simulink model "PMSM_CascadedMPC"  (R2025b)
settings: Solver=ode3  StartTime=0.0  StopTime=12  FixedStep=5e-6  MaxStep=1e-4  RelTol=1e-3
PreLoadFcn:
  | run('params_pmsm_inverter')
undefined symbols (not defined in the file): B_fric, J, Ld, Lq, pp, PsiPM, Rs, Ts_ctrl, Ts_sim, Vdc
libraries: nesl_utility x16, fl_lib x11, ee_lib x8, simulink x1, sdl_lib x1
(part 1 of 2)
settings Model: SimulationMode=accelerator  Creator=Harish  LastModifiedBy=Harish

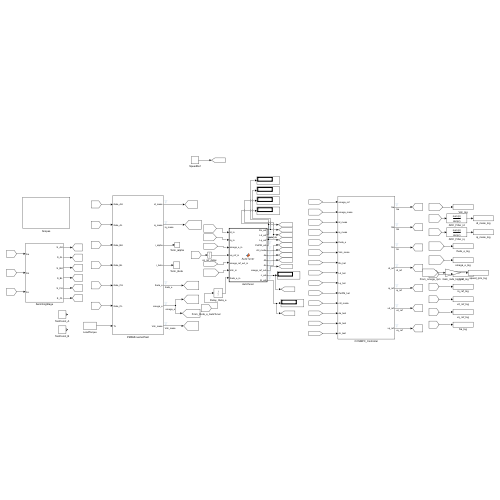
[thumbnail: Simulink's stored preview of the top-level diagram]
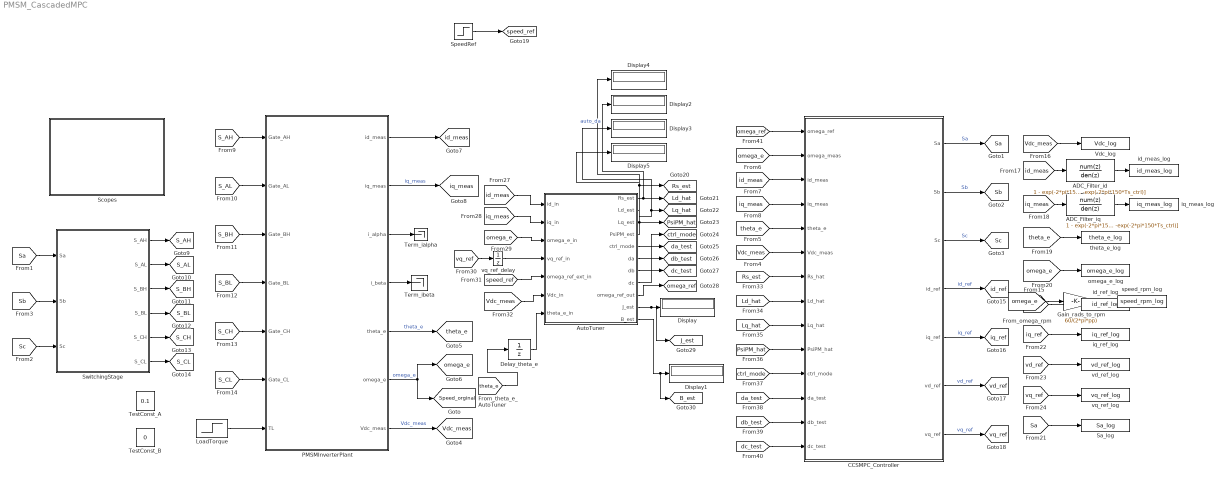
== system PMSM_CascadedMPC ==
  ADC_Filter_id : DiscreteFilter  Numerator=1 - exp(-2*pi*150*Ts_ctrl)  Denominator=[1, -exp(-2*pi*150*Ts_ctrl)]  SampleTime=Ts_ctrl
  ADC_Filter_iq : DiscreteFilter  Numerator=1 - exp(-2*pi*150*Ts_ctrl)  Denominator=[1, -exp(-2*pi*150*Ts_ctrl)]  SampleTime=Ts_ctrl
  AutoTuner : MATLAB Function  TreatAsAtomicUnit=on
  CCSMPC_Controller : Subsystem
  Delay_theta_e : UnitDelay  SampleTime=1e-4  HasFrameUpgradeWarning=on
  Display{,1..5} (6 alike) : Display
  Gain_rads_to_rpm : Gain  Gain=60/(2*pi*pp)
  LoadTorque : Step  Time=6.1  After=-250  SampleTime=0
  PMSMInverterPlant : Subsystem
  Sa_log : ToWorkspace  VariableName=Sa_log  SaveFormat=Timeseries  SampleTime=-1
  Scopes : Subsystem
  SpeedRef : Step  Time=6.1  After=800  SampleTime=0
  SwitchingStage : Subsystem
  Term_ialpha : Terminator
  Term_ibeta : Terminator
  TestConst_A : Constant  Value=0.1
  TestConst_B : Constant  Value=0
  Vdc_log : ToWorkspace  VariableName=Vdc_log  SaveFormat=Timeseries  SampleTime=-1
  id_meas_log : ToWorkspace  VariableName=id_meas_log  SaveFormat=Timeseries  SampleTime=-1
  id_ref_log : ToWorkspace  VariableName=id_ref_log  SaveFormat=Timeseries  SampleTime=-1
  iq_meas_log : ToWorkspace  VariableName=iq_meas_log  SaveFormat=Timeseries  SampleTime=-1
  iq_ref_log : ToWorkspace  VariableName=iq_ref_log  SaveFormat=Timeseries  SampleTime=-1
  omega_e_log : ToWorkspace  VariableName=omega_e_log  SaveFormat=Timeseries  SampleTime=-1
  speed_rpm_log : ToWorkspace  VariableName=speed_rpm_log  SaveFormat=Timeseries  SampleTime=-1
  theta_e_log : ToWorkspace  VariableName=theta_e_log  SaveFormat=Timeseries  SampleTime=-1
  vd_ref_log : ToWorkspace  VariableName=vd_ref_log  SaveFormat=Timeseries  SampleTime=-1
  vq_ref_delay : UnitDelay  SampleTime=-1  HasFrameUpgradeWarning=on
  vq_ref_log : ToWorkspace  VariableName=vq_ref_log  SaveFormat=Timeseries  SampleTime=-1
  tag scope: B_est=global, J_est=global, Ld_hat=global, Lq_hat=global, PsiPM_hat=global, Rs_est=global, S_AH=global, S_AL=global, S_BH=global, S_BL=global, S_CH=global, S_CL=global, Sa=global, Sb=global, Sc=global, Speed_orginal=global, Vdc_meas=global, ctrl_mode=global, da_test=global, db_test=global, dc_test=global, id_meas=global, id_ref=global, iq_meas=global, iq_ref=global, omega_e=global, omega_ref=global, speed_ref=global, theta_e=global, vd_ref=global, vq_ref=global
  wires:
  PMSMInverterPlant/6(omega_e) -> [Speed_orginal], [omega_e]  "omega_e"
  PMSMInverterPlant/1(id_meas) -> [id_meas]
  PMSMInverterPlant/2(iq_meas) -> [iq_meas]  "iq_meas"
  PMSMInverterPlant/5(theta_e) -> [theta_e]  "theta_e"
  LoadTorque/1 -> PMSMInverterPlant/7(TL)
  PMSMInverterPlant/3(i_alpha) -> Term_ialpha/1
  PMSMInverterPlant/4(i_beta) -> Term_ibeta/1
  [Sa] -> SwitchingStage/1(Sa)
  [Sb] -> SwitchingStage/2(Sb)
  [Sc] -> SwitchingStage/3(Sc)
  PMSMInverterPlant/7(Vdc_meas) -> [Vdc_meas]  "Vdc_meas"
  SwitchingStage/1(S_AH) -> [S_AH]
  SwitchingStage/2(S_AL) -> [S_AL]
  SwitchingStage/3(S_BH) -> [S_BH]
  SwitchingStage/4(S_BL) -> [S_BL]
  SwitchingStage/5(S_CH) -> [S_CH]
  SwitchingStage/6(S_CL) -> [S_CL]
  [S_AH] -> PMSMInverterPlant/1(Gate_AH)
  [S_AL] -> PMSMInverterPlant/2(Gate_AL)
  [S_BH] -> PMSMInverterPlant/3(Gate_BH)
  [S_BL] -> PMSMInverterPlant/4(Gate_BL)
  [S_CH] -> PMSMInverterPlant/5(Gate_CH)
  [S_CL] -> PMSMInverterPlant/6(Gate_CL)
  [Vdc_meas] -> Vdc_log/1
  [theta_e] -> theta_e_log/1
  [omega_e] -> omega_e_log/1
  [Sa] -> Sa_log/1
  [id_ref] -> id_ref_log/1
  [iq_ref] -> iq_ref_log/1
  [vd_ref] -> vd_ref_log/1
  [vq_ref] -> vq_ref_log/1
  [omega_e] -> CCSMPC_Controller/2(omega_meas)
  [id_meas] -> CCSMPC_Controller/3(id_meas)
  [iq_meas] -> CCSMPC_Controller/4(iq_meas)
  [Vdc_meas] -> CCSMPC_Controller/6(Vdc_meas)
  [theta_e] -> CCSMPC_Controller/5(theta_e)
  [dc_test] -> CCSMPC_Controller/14(dc_test)
  [db_test] -> CCSMPC_Controller/13(db_test)
  [da_test] -> CCSMPC_Controller/12(da_test)
  [ctrl_mode] -> CCSMPC_Controller/11(ctrl_mode)
  [PsiPM_hat] -> CCSMPC_Controller/10(PsiPM_hat)
  [Lq_hat] -> CCSMPC_Controller/9(Lq_hat)
  [Ld_hat] -> CCSMPC_Controller/8(Ld_hat)
  [Rs_est] -> CCSMPC_Controller/7(Rs_hat)
  CCSMPC_Controller/1(Sa) -> [Sa]  "Sa"
  CCSMPC_Controller/2(Sb) -> [Sb]  "Sb"
  CCSMPC_Controller/3(Sc) -> [Sc]  "Sc"
  CCSMPC_Controller/4(id_ref) -> [id_ref]  "id_ref"
  CCSMPC_Controller/5(iq_ref) -> [iq_ref]  "iq_ref"
  CCSMPC_Controller/6(vd_ref) -> [vd_ref]  "vd_ref"
  CCSMPC_Controller/7(vq_ref) -> [vq_ref]  "vq_ref"
  SpeedRef/1 -> [speed_ref]
  [vq_ref] -> vq_ref_delay/1
  AutoTuner/1(Rs_est) -> Display4/1, [Rs_est]
  AutoTuner/2(Ld_est) -> Display2/1, [Ld_hat]  "auto_da"
  AutoTuner/3(Lq_est) -> Display3/1, [Lq_hat]
  AutoTuner/4(PsiPM_est) -> Display5/1, [PsiPM_hat]
  [omega_ref] -> CCSMPC_Controller/1(omega_ref)
  AutoTuner/5(ctrl_mode) -> [ctrl_mode]
  AutoTuner/6(da) -> [da_test]
  AutoTuner/7(db) -> [db_test]
  AutoTuner/8(dc) -> [dc_test]
  AutoTuner/9(omega_ref_out) -> [omega_ref]
  [theta_e] -> Delay_theta_e/1
  Delay_theta_e/1 -> AutoTuner/7(theta_e_in)
  [Vdc_meas] -> AutoTuner/6(Vdc_in)
  [speed_ref] -> AutoTuner/5(omega_ref_ext_in)
  vq_ref_delay/1 -> AutoTuner/4(vq_ref_in)
  [omega_e] -> AutoTuner/3(omega_e_in)
  [iq_meas] -> AutoTuner/2(iq_in)
  [id_meas] -> AutoTuner/1(id_in)
  AutoTuner/11(B_est) -> [B_est], Display1/1
  AutoTuner/10(J_est) -> [J_est], Display/1
  [omega_e] -> Gain_rads_to_rpm/1
  Gain_rads_to_rpm/1 -> speed_rpm_log/1
  [id_meas] -> ADC_Filter_id/1
  ADC_Filter_id/1 -> id_meas_log/1
  [iq_meas] -> ADC_Filter_iq/1
  ADC_Filter_iq/1 -> iq_meas_log/1

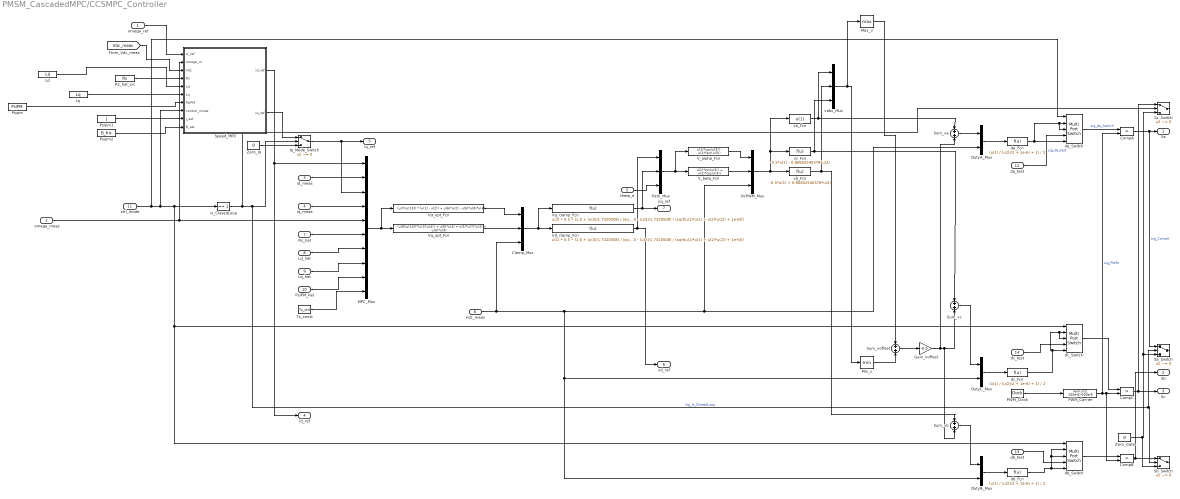
== system PMSM_CascadedMPC/CCSMPC_Controller ==
  omega_ref : Inport  SampleTime=Ts_ctrl
  omega_meas : Inport  Port=2  SampleTime=Ts_ctrl
  id_meas : Inport  Port=3  SampleTime=Ts_ctrl
  iq_meas : Inport  Port=4  SampleTime=Ts_ctrl
  theta_e : Inport  Port=5  SampleTime=Ts_ctrl
  Vdc_meas : Inport  Port=6  SampleTime=Ts_ctrl
  Rs_hat : Inport  Port=7  SampleTime=Ts_ctrl
  Ld_hat : Inport  Port=8  SampleTime=Ts_ctrl
  Lq_hat : Inport  Port=9  SampleTime=Ts_ctrl
  PsiPM_hat : Inport  Port=10  SampleTime=Ts_ctrl
  ctrl_mode : Inport  Port=11  SampleTime=Ts_ctrl
  da_test : Inport  Port=12
  db_test : Inport  Port=13
  dc_test : Inport  Port=14
  Clamp_Mux : Mux  Inputs=3
  CompA : RelationalOperator  Operator=>  OutDataTypeStr=boolean  SampleTime=Ts_sim  RndMeth=Simplest  InputSameDT=off
  CompB : RelationalOperator  Operator=>  OutDataTypeStr=boolean  SampleTime=Ts_sim  RndMeth=Simplest  InputSameDT=off
  CompC : RelationalOperator  Operator=>  OutDataTypeStr=boolean  SampleTime=Ts_sim  RndMeth=Simplest  InputSameDT=off
  DutyA_Mux : Mux  Inputs=2
  DutyB_Mux : Mux  Inputs=2
  DutyC_Mux : Mux  Inputs=2
  Gain_voffset : Gain  Gain=-0.5
  Iq_Mode_Switch : Switch  Criteria=u2 ~= 0  Threshold=0.5  SaturateOnIntegerOverflow=off  InputSameDT=off
  Is_ClosedLoop : simulink/Logic and Bit Operations/Compare To Constant  relop===  const=1  OutDataTypeStr=boolean
  Ld : Constant  Value=Ld
  Lq : Constant  Value=Lq
  MPC_Mux : Mux  Inputs=10
  Max_v : MinMax  Function=max
  Min_v : MinMax
  PWM_Carrier : Fcn  Expr=rem(u(1), 100e-6)/100e-6
  PWM_Clock : DigitalClock  SampleTime=Ts_sim
  Park_Mux : Mux  Inputs=3
  Psipm : Constant  Value=PsiPM
  Psipm1 : Constant  Value=J
  Psipm2 : Constant  Value=B_fric
  Rs_hat_src : Constant  Value=Rs
  SVPWM_Mux : Mux  Inputs=3
  Sa_Switch : Switch  Criteria=u2 ~= 0  Threshold=0.5  SaturateOnIntegerOverflow=off  InputSameDT=off
  Sb_Switch : Switch  Criteria=u2 ~= 0  Threshold=0.5  SaturateOnIntegerOverflow=off  InputSameDT=off
  Sc_Switch : Switch  Criteria=u2 ~= 0  Threshold=0.5  SaturateOnIntegerOverflow=off  InputSameDT=off
  Speed_MPC : MATLAB Function  TreatAsAtomicUnit=on
  Sum_va : Sum
  Sum_vb : Sum
  Sum_vc : Sum
  Sum_voffset : Sum
  Ts_const : Constant  Value=Ts_ctrl  SampleTime=Ts_ctrl
  V_alpha_Fcn : Fcn  Expr=u(1)*cos(u(3)) - u(2)*sin(u(3))
  V_beta_Fcn : Fcn  Expr=u(1)*sin(u(3)) + u(2)*cos(u(3))
  Vd_clamp_Fcn : Fcn  Expr=u(1) * 0.5 * (1.0 + (u(3)/1.7320508) / (sqrt(u(1)*u(1) + u(2)*u(2)) + 1e-6) - abs(1.0 - (u(3)/1.7320508) / (sqrt(u(1)*u(1) + u(2)*u(2)) + 1e-6)))
  Vd_opt_Fcn : Fcn  Expr=(u(7)/u(10)) * (u(1) - u(2)) + u(6)*u(2) - u(5)*u(8)*u(4);
  Vq_clamp_Fcn : Fcn  Expr=u(2) * 0.5 * (1.0 + (u(3)/1.7320508) / (sqrt(u(1)*u(1) + u(2)*u(2)) + 1e-6) - abs(1.0 - (u(3)/1.7320508) / (sqrt(u(1)*u(1) + u(2)*u(2)) + 1e-6)))
  Vq_opt_Fcn : Fcn  Expr=(u(8)/u(10))*(u(3)-u(4)) + u(6)*u(4) + u(5)*u(7)*u(2) + u(5)*u(9)
  Zero_Gate : Constant  Value=0  OutDataTypeStr=boolean  SampleTime=Ts_ctrl
  Zero_Iq : Constant  Value=0  SampleTime=Ts_ctrl
  da_Fcn : Fcn  Expr=(u(1) / (u(2)/2 + 1e-6) + 1) / 2
  da_Switch : MultiPortSwitch  DataPortOrder=Zero-based contiguous  Inputs=4  DataPortIndices={1,4,2}  zeroidx=on  SaturateOnIntegerOverflow=off  InputSameDT=off
  db_Fcn : Fcn  Expr=(u(1) / (u(2)/2 + 1e-6) + 1) / 2
  db_Switch : MultiPortSwitch  DataPortOrder=Zero-based contiguous  Inputs=4  DataPortIndices={1,4,2}  zeroidx=on  SaturateOnIntegerOverflow=off  InputSameDT=off
  dc_Fcn : Fcn  Expr=(u(1) / (u(2)/2 + 1e-6) + 1) / 2
  dc_Switch : MultiPortSwitch  DataPortOrder=Zero-based contiguous  Inputs=4  DataPortIndices={1,4,2}  zeroidx=on  SaturateOnIntegerOverflow=off  InputSameDT=off
  va_Fcn : Fcn  Expr=u(1)
  vabc_Mux : Mux  Inputs=3
  vb_Fcn : Fcn  Expr=-0.5*u(1) + 0.86602540378*u(2)
  vc_Fcn : Fcn  Expr=-0.5*u(1) - 0.86602540378*u(2)
  Sa : Outport  SampleTime=Ts_ctrl
  Sb : Outport  Port=2  SampleTime=Ts_ctrl
  Sc : Outport  Port=3  SampleTime=Ts_ctrl
  id_ref : Outport  Port=4  SampleTime=Ts_ctrl
  iq_ref : Outport  Port=5  SampleTime=Ts_ctrl
  vd_ref : Outport  Port=6  SampleTime=Ts_ctrl
  vq_ref : Outport  Port=7  SampleTime=Ts_ctrl
  wires:
  Min_v/1 -> Sum_voffset/2
  SVPWM_Mux/1 -> va_Fcn/1, vc_Fcn/1, vb_Fcn/1
  omega_meas/1 -> Speed_MPC/2(omega_m), MPC_Mux/5
  Ld/1 -> Speed_MPC/5(Ld)
  db_Switch/1 -> CompB/1
  [Vdc_meas] -> Speed_MPC/3(Vdc)
  Park_Mux/1 -> V_alpha_Fcn/1, V_beta_Fcn/1
  Iq_Mode_Switch/1 -> MPC_Mux/3, iq_ref/1
  Rs_hat_src/1 -> Speed_MPC/4(Rs)
  Sum_va/1 -> DutyA_Mux/1
  Vq_opt_Fcn/1 -> Clamp_Mux/2
  Lq/1 -> Speed_MPC/6(Lq)
  Zero_Gate/1 -> Sa_Switch/3, Sc_Switch/3, Sb_Switch/3
  V_beta_Fcn/1 -> SVPWM_Mux/2
  Psipm/1 -> Speed_MPC/7(PsiPM)
  Vd_opt_Fcn/1 -> Clamp_Mux/1
  ctrl_mode/1 -> dc_Switch/1, db_Switch/1, Is_ClosedLoop/1, Speed_MPC/8(control_mode), da_Switch/1
  Speed_MPC/1(id_ref) -> MPC_Mux/1, id_ref/1
  Vd_clamp_Fcn/1 -> vd_ref/1, Park_Mux/1
  Speed_MPC/2(iq_ref) -> Iq_Mode_Switch/1
  Zero_Iq/1 -> Iq_Mode_Switch/3
  id_meas/1 -> MPC_Mux/2
  Is_ClosedLoop/1 -> Sb_Switch/2, Sa_Switch/2, Iq_Mode_Switch/2, Sc_Switch/2  "sig_Is_ClosedLoop"
  iq_meas/1 -> MPC_Mux/4
  Gain_voffset/1 -> Sum_vb/2, Sum_vc/2, Sum_va/2
  Rs_hat/1 -> MPC_Mux/6
  da_test/1 -> da_Switch/4  "sig_da_test"
  Ld_hat/1 -> MPC_Mux/7
  db_test/1 -> db_Switch/4
  Clamp_Mux/1 -> Vd_clamp_Fcn/1, Vq_clamp_Fcn/1
  Lq_hat/1 -> MPC_Mux/8
  PsiPM_hat/1 -> MPC_Mux/9
  dc_test/1 -> dc_Switch/4
  Ts_const/1 -> MPC_Mux/10
  MPC_Mux/1 -> Vq_opt_Fcn/1, Vd_opt_Fcn/1
  Vdc_meas/1 -> DutyC_Mux/2, DutyB_Mux/2, DutyA_Mux/2, SVPWM_Mux/3, Clamp_Mux/3
  theta_e/1 -> Park_Mux/3
  dc_Fcn/1 -> dc_Switch/5, dc_Switch/3, dc_Switch/2
  Vq_clamp_Fcn/1 -> Park_Mux/2, vq_ref/1
  V_alpha_Fcn/1 -> SVPWM_Mux/1
  da_Switch/1 -> CompA/1  "sig_da_Switch"
  va_Fcn/1 -> Sum_va/1, vabc_Mux/1
  vc_Fcn/1 -> Sum_vc/1, vabc_Mux/3
  vb_Fcn/1 -> Sum_vb/1, vabc_Mux/2
  vabc_Mux/1 -> Min_v/1, Max_v/1
  Max_v/1 -> Sum_voffset/1
  Sum_voffset/1 -> Gain_voffset/1
  Sum_vc/1 -> DutyC_Mux/1
  DutyC_Mux/1 -> dc_Fcn/1
  Sum_vb/1 -> DutyB_Mux/1
  DutyA_Mux/1 -> da_Fcn/1
  CompA/1 -> Sa/1, Sa_Switch/1  "sig_CompA"
  DutyB_Mux/1 -> db_Fcn/1
  da_Fcn/1 -> da_Switch/5, da_Switch/3, da_Switch/2
  PWM_Clock/1 -> PWM_Carrier/1
  CompC/1 -> Sc_Switch/1, Sc/1
  db_Fcn/1 -> db_Switch/5, db_Switch/2, db_Switch/3
  dc_Switch/1 -> CompC/1
  PWM_Carrier/1 -> CompB/2, CompC/2, CompA/2  "sig_PWM"
  CompB/1 -> Sb/1, Sb_Switch/1
  omega_ref/1 -> Speed_MPC/1(w_ref)
  Psipm1/1 -> Speed_MPC/9(J_est)
  Psipm2/1 -> Speed_MPC/10(B_est)

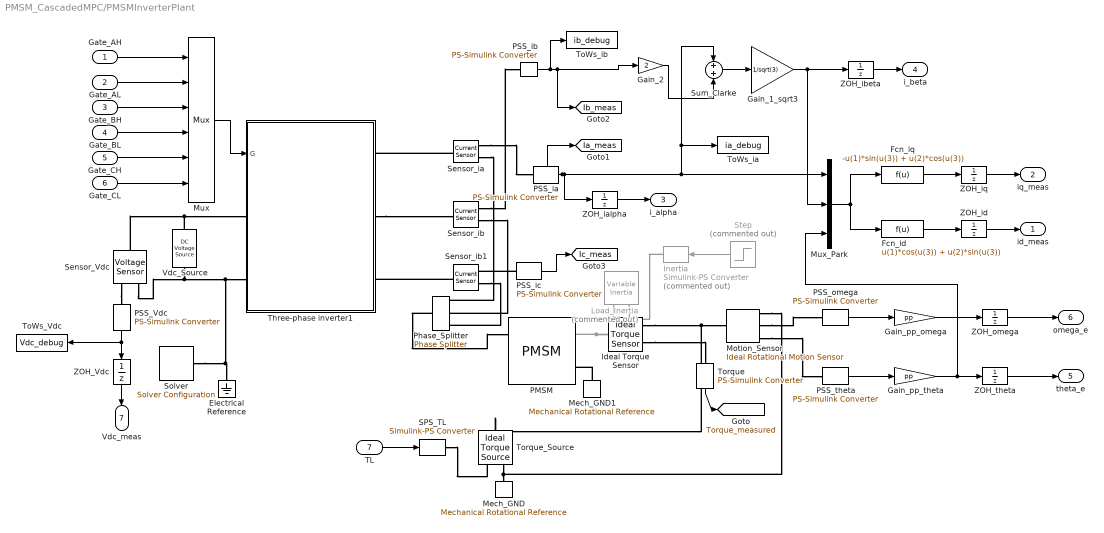
== system PMSM_CascadedMPC/PMSMInverterPlant ==
  Gate_AH : Inport
  Gate_AL : Inport  Port=2
  Gate_BH : Inport  Port=3
  Gate_BL : Inport  Port=4
  Gate_CH : Inport  Port=5
  Gate_CL : Inport  Port=6
  TL : Inport  Port=7
  Electrical Reference : fl_lib/Electrical/Electrical Elements/Electrical Reference
  Fcn_id : Fcn  Expr=u(1)*cos(u(3)) + u(2)*sin(u(3))
  Fcn_iq : Fcn  Expr=-u(1)*sin(u(3)) + u(2)*cos(u(3))
  Gain_1_sqrt3 : Gain  Gain=1/sqrt(3)
  Gain_2 : Gain  Gain=2
  Gain_pp_omega : Gain  Gain=pp
  Gain_pp_theta : Gain  Gain=pp
  Ideal Torque Sensor : fl_lib/Mechanical/Mechanical Sensors/Ideal Torque Sensor
  Inertia : nesl_utility/Simulink-PS Converter  Commented=on  PhysicalDomain=network_engine_domain  SubClassName=ps_input  LeftPortType=input  RightPortType=output  PseudoPeriodic=off  Frequencies=[]  NoiseDistribution=none  NoiseParameters=[]  Unit=1  AffineConversion=off  FilteringAndDerivatives=filter  SimscapeFilterOrder=1  InputFilterTimeConstant=0.001  UdotUserProvided=0
  Load_Inertia : sdl_lib/Inertias & Loads/Variable Inertia  Commented=on  minimum_inertia=0.0001 kg*m^2  L_specify=off  L_priority=High  L=0 kg*m^2/s  L_nominal_specify=off  L_nominal_value=1  L_nominal_unit=kg*m^2/s
      settings: InternalSimscapePortConfiguration="{\"Bottom\":[],\"Left\":[{\"id\":\"I\",\"label\":\"\",\"type\":\"input\"},{\"id\":\"A\",\"label\":\"\",\"type\":\"foundation.mechanical.rotational.rotational\"}],\"Right\":[],\"Top\":[]}"
  Mech_GND : fl_lib/Mechanical/Rotational Elements/Mechanical Rotational Reference
  Mech_GND1 : fl_lib/Mechanical/Rotational Elements/Mechanical Rotational Reference
  Motion_Sensor : fl_lib/Mechanical/Mechanical Sensors/Ideal Rotational Motion Sensor  reference=foundation.enum.MeasurementReference.difference  acceleration_port=false  velocity_port=true  position_port=true  wrap_angle=false  offset=0 rad
  Mux : Mux  Inputs=6
  Mux_Park : Mux  Inputs=3
  PMSM : ee_lib/Electromechanical/Permanent Magnet/PMSM  port_option=1  winding_type=ee.enum.electromech.statorconfiguration.wye  machine_param=ee.enum.pmsm.parameterization.constant  nPolePairs=pp  pmflux_param=ee.enum.pmflux.fluxlinkage  pm_flux_linkage=PsiPM Wb  torque_constant=0.18 N*m/A  back_emf_constant=0.18 V*s/rad  stator_param=1  Ld=Ld H  Lq=Lq H  idVec=[-200, 0, 200] A  iqVec=[-200, 0, 200] A  LdMatrix=0.0002 * ones(3, 3) H  LqMatrix=0.0002 * ones(3, 3) H  PmMatrix=0.1 * ones(3, 3) Wb  ktMatrix=0.18 * ones(3, 3) N*m/A  keMatrix=0.18 * ones(3, 3) V*s/rad  L0=0.00016 H  Ls=0.0002 H  Lm=-0.00002 H  Ms=0.00002 H  Rs=Rs Ohm  zero_sequence=ee.enum.park.zerosequence.include  axes_param=ee.enum.rotorangle.daxis  loss_param=ee.enum.ironloss.none  losses_oc=[0, 0, 0] W  losses_sc=[0, 0, 0] W  f_losses=60 Hz  Isc_losses=95 A  J=J kg*m^2  lam=B_fric N*m*s/rad  i_d_specify=off  i_d_priority=None  i_d=0 A  i_d_nominal_specify=off  i_d_nominal_value=1  i_d_nominal_unit=A  i_q_specify=off  i_q_priority=None  i_q=0 A  i_q_nominal_specify=off  i_q_nominal_value=1  i_q_nominal_unit=A  torque_specify=off  torque_priority=None  torque=0 N*m  torque_nominal_specify=off  torque_nominal_value=1  torque_nominal_unit=N*m  angular_velocity_specify=off  angular_velocity_priority=High  angular_velocity=0 rpm  angular_velocity_nominal_specify=off  angular_velocity_nominal_value=1  angular_velocity_nominal_unit=rpm  angular_position_specify=off  angular_position_priority=High  angular_position=0 deg  angular_position_nominal_specify=off  angular_position_nominal_value=1  angular_position_nominal_unit=deg  alpha=3.93e-3 1/K  alpha_flux=-0.001 1/K  Tmeas=298.15 K  stator_thermal_mass=100 J/K  rotor_thermal_mass=200 J/K  Rm_percent_rotor=90  Rd_percent_rotor=30  temperatureA_specify=off  temperatureA_priority=High  temperatureA=25 degC  temperatureA_nominal_specify=off  temperatureA_nominal_value=1  temperatureA_nominal_unit=degC  temperatureB_specify=off  temperatureB_priority=High  temperatureB=25 degC  temperatureB_nominal_specify=off  temperatureB_nominal_value=1  temperatureB_nominal_unit=degC  temperatureC_specify=off  temperatureC_priority=High  temperatureC=25 degC  temperatureC_nominal_specify=off  temperatureC_nominal_value=1  temperatureC_nominal_unit=degC  temperatureR_specify=off  temperatureR_priority=High  temperatureR=25 degC  temperatureR_nominal_specify=off  temperatureR_nominal_value=1  temperatureR_nominal_unit=degC
      settings: InternalSimscapePortConfiguration="{\"Bottom\":[],\"Left\":[{\"id\":\"N\",\"label\":\"~\",\"type\":\"foundation.electrical.three_phase\"},{\"id\":\"n\",\"label\":\"n\",\"type\":\"foundation.electrical.electrical\"}],\"Right\":[{\"id\":\"R\",\"label\":\"R\",\"type\":\"foundation.mechanical.rotational.rotational\"},{\"id\":\"C\",\"label\":\"C\",\"type\":\"foundation.mechanical.rotational.rotational\"}],\"Top\":[]}"
  PSS_Vdc : nesl_utility/PS-Simulink Converter  PhysicalDomain=network_engine_domain  SubClassName=ps_output  LeftPortType=input  RightPortType=output  PseudoPeriodic=off  Frequencies=[]  VectorFormat=inherit  Unit=inherit  AffineConversion=off
  PSS_ia : nesl_utility/PS-Simulink Converter  PhysicalDomain=network_engine_domain  SubClassName=ps_output  LeftPortType=input  RightPortType=output  PseudoPeriodic=off  Frequencies=[]  VectorFormat=inherit  Unit=inherit  AffineConversion=off
  PSS_ib : nesl_utility/PS-Simulink Converter  PhysicalDomain=network_engine_domain  SubClassName=ps_output  LeftPortType=input  RightPortType=output  PseudoPeriodic=off  Frequencies=[]  VectorFormat=inherit  Unit=inherit  AffineConversion=off
  PSS_ic : nesl_utility/PS-Simulink Converter  PhysicalDomain=network_engine_domain  SubClassName=ps_output  LeftPortType=input  RightPortType=output  PseudoPeriodic=off  Frequencies=[]  VectorFormat=inherit  Unit=inherit  AffineConversion=off
  PSS_omega : nesl_utility/PS-Simulink Converter  PhysicalDomain=network_engine_domain  SubClassName=ps_output  LeftPortType=input  RightPortType=output  PseudoPeriodic=off  Frequencies=[]  VectorFormat=inherit  Unit=inherit  AffineConversion=off
  PSS_theta : nesl_utility/PS-Simulink Converter  PhysicalDomain=network_engine_domain  SubClassName=ps_output  LeftPortType=input  RightPortType=output  PseudoPeriodic=off  Frequencies=[]  VectorFormat=inherit  Unit=inherit  AffineConversion=off
  Phase_Splitter : ee_lib/Connectors & References/Phase Splitter
  SPS_TL : nesl_utility/Simulink-PS Converter  PhysicalDomain=network_engine_domain  SubClassName=ps_input  LeftPortType=input  RightPortType=output  PseudoPeriodic=off  Frequencies=[]  NoiseDistribution=none  NoiseParameters=[]  Unit=1  AffineConversion=off  FilteringAndDerivatives=filter  SimscapeFilterOrder=1  InputFilterTimeConstant=0.001  UdotUserProvided=0
  Sensor_Vdc : fl_lib/Electrical/Electrical Sensors/Voltage Sensor
  Sensor_ia : fl_lib/Electrical/Electrical Sensors/Current Sensor
  Sensor_ib : fl_lib/Electrical/Electrical Sensors/Current Sensor
  Sensor_ib1 : fl_lib/Electrical/Electrical Sensors/Current Sensor
  Solver : nesl_utility/Solver Configuration  PhysicalDomain=network_engine_domain  SubClassName=solver  LeftPortType=input  RightPortType=generic  Tones=[]  Harmonics=[]  SimulateNoise=off  Profile=off  UseLocalSampling=off  EnableSwitchedLinearOptims=on  FrequencyDomain=off  UseCCode=off  RelTol=0.001  AbsTol=0.001  MinStep=1e-09  ToWorkspace=off  RevertToSquareIcSolve=off  NumHomotopyIterations=100  PhasorMode=off  PhasorModeNumHarmonics=1  ConsistencySolver=NEWTON_XTOL_AFTER_FTOL  IndexReductionMethod=DerivativeReplacement  DoDC=off  ResidualTolerance=1e-09  ConsistencyTolSource=GLOBAL  ConsistencyAbsTol=0.001  ConsistencyRelTol=0.001  ConsistencyTolFactor=0.001  UseLocalSolver=on  LocalSolverChoice=NE_BACKWARD_EULER_ADVANCER  ResolveIndetEquations=on  FunctionEvalNumThread=1  LocalSolverSampleTime=Ts_sim  DoFixedCost=off  MaxNonlinIter=3  MaxModeIter=2  ComputeImpulses=off  ImpulseIterations=2  LinearAlgebra=auto  LinearAlgebraNumThread=0  EquationFormulation=NE_TIME_EF  DelaysMemoryBudget=1024  AutomaticFiltering=on  FilteringTimeConstant=0.001  PartitionStorageMethod=AS_NEEDED  PartitionMemoryBudget=1024  PartitionMethod=ROBUST  MultibodyUseLocalSolver=off  MultibodyLocalSolverChoice=ODE1  MultibodyLocalSolverSampleTime=0.001
  Step : Step  Commented=on  Time=12  After=0.5  SampleTime=0
  Sum_Clarke : Sum
  Three-phase inverter1 : Subsystem
      mask Display: image('Inverter.jpg');
  ToWs_Vdc : ToWorkspace  VariableName=Vdc_debug  SampleTime=-1
  ToWs_ia : ToWorkspace  VariableName=ia_debug  SampleTime=-1
  ToWs_ib : ToWorkspace  VariableName=ib_debug  SampleTime=-1
  Torque : nesl_utility/PS-Simulink Converter  PhysicalDomain=network_engine_domain  SubClassName=ps_output  LeftPortType=input  RightPortType=output  PseudoPeriodic=off  Frequencies=[]  VectorFormat=inherit  Unit=inherit  AffineConversion=off
  Torque_Source : fl_lib/Mechanical/Mechanical Sources/Ideal Torque Source
  Vdc_Source : fl_lib/Electrical/Electrical Sources/DC Voltage Source  v0=Vdc V
  ZOH_Vdc : UnitDelay  InitialCondition=Vdc  SampleTime=Ts_ctrl  HasFrameUpgradeWarning=on
  ZOH_ialpha : UnitDelay  SampleTime=Ts_ctrl  HasFrameUpgradeWarning=on
  ZOH_ibeta : UnitDelay  SampleTime=Ts_ctrl  HasFrameUpgradeWarning=on
  ZOH_id : UnitDelay  SampleTime=Ts_ctrl  HasFrameUpgradeWarning=on
  ZOH_iq : UnitDelay  SampleTime=Ts_ctrl  HasFrameUpgradeWarning=on
  ZOH_omega : UnitDelay  SampleTime=Ts_ctrl  HasFrameUpgradeWarning=on
  ZOH_theta : UnitDelay  SampleTime=Ts_ctrl  HasFrameUpgradeWarning=on
  id_meas : Outport
  iq_meas : Outport  Port=2
  i_alpha : Outport  Port=3
  i_beta : Outport  Port=4
  theta_e : Outport  Port=5
  omega_e : Outport  Port=6
  Vdc_meas : Outport  Port=7
  tag scope: Ia_meas=global, Ib_meas=global, Ic_meas=global, Torque_measured=global
  wires:
  TL/1 -> SPS_TL/1
  Mux_Park/1 -> Fcn_iq/1, Fcn_id/1
  PSS_omega/1 -> Gain_pp_omega/1
  Fcn_iq/1 -> ZOH_iq/1
  Gain_2/1 -> Sum_Clarke/2
  PSS_theta/1 -> Gain_pp_theta/1
  Fcn_id/1 -> ZOH_id/1
  Gain_1_sqrt3/1 -> ZOH_ibeta/1, Mux_Park/2
  PSS_Vdc/1 -> ZOH_Vdc/1, ToWs_Vdc/1
  PSS_ia/1 -> [Ia_meas], ToWs_ia/1, Sum_Clarke/1, Mux_Park/1, ZOH_ialpha/1
  Gain_pp_omega/1 -> ZOH_omega/1
  Gain_pp_theta/1 -> ZOH_theta/1, Mux_Park/3
  ZOH_Vdc/1 -> Vdc_meas/1
  ZOH_omega/1 -> omega_e/1
  ZOH_theta/1 -> theta_e/1
  PSS_ib/1 -> [Ib_meas], Gain_2/1, ToWs_ib/1
  Sum_Clarke/1 -> Gain_1_sqrt3/1
  ZOH_ialpha/1 -> i_alpha/1
  ZOH_ibeta/1 -> i_beta/1
  ZOH_iq/1 -> iq_meas/1
  ZOH_id/1 -> id_meas/1
  Gate_AH/1 -> Mux/1
  Gate_AL/1 -> Mux/2
  Gate_BH/1 -> Mux/3
  Gate_BL/1 -> Mux/4
  Gate_CH/1 -> Mux/5
  Gate_CL/1 -> Mux/6
  Mux/1 -> Three-phase inverter1/1(G)
  Step/1 -> Inertia/1
  Torque/1 -> [Torque_measured]
  PSS_ic/1 -> [Ic_meas]
  connections:
  SPS_TL/RConn1 -- Torque_Source/RConn1
  Torque_Source/RConn2 -- Motion_Sensor/RConn1 -- Mech_GND/LConn1
  Load_Inertia/LConn2 -- Ideal Torque Sensor/LConn1 -- PMSM/RConn1
  Phase_Splitter/LConn1 -- PMSM/LConn1
  Motion_Sensor/RConn2 -- PSS_omega/LConn1
  Motion_Sensor/RConn3 -- PSS_theta/LConn1
  Sensor_ib/RConn1 -- PSS_ib/LConn1
  Sensor_Vdc/RConn1 -- PSS_Vdc/LConn1
  Sensor_ib/RConn2 -- Phase_Splitter/RConn2
  Sensor_ia/RConn1 -- PSS_ia/LConn1
  Sensor_ia/RConn2 -- Phase_Splitter/RConn1
  Vdc_Source/LConn1 -- Sensor_Vdc/LConn1 -- Three-phase inverter1/LConn1
  Vdc_Source/RConn1 -- Three-phase inverter1/LConn2 -- Solver/RConn1 -- Electrical Reference/LConn1 -- Sensor_Vdc/RConn2
  Sensor_ia/LConn1 -- Three-phase inverter1/RConn1
  Three-phase inverter1/RConn2 -- Sensor_ib/LConn1
  Inertia/RConn1 -- Load_Inertia/LConn1
  Mech_GND1/LConn1 -- PMSM/RConn2
  Ideal Torque Sensor/RConn1 -- Torque_Source/LConn1 -- Motion_Sensor/LConn1
  Ideal Torque Sensor/RConn2 -- Torque/LConn1
  Sensor_ib1/LConn1 -- Three-phase inverter1/RConn3
  Sensor_ib1/RConn2 -- Phase_Splitter/RConn3
  PSS_ic/LConn1 -- Sensor_ib1/RConn1

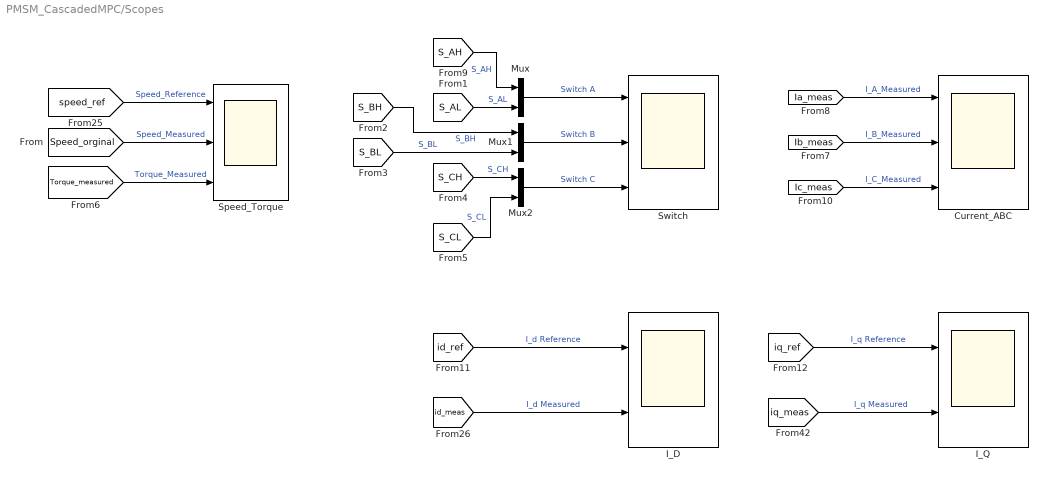
== system PMSM_CascadedMPC/Scopes ==
  Current_ABC : Scope  NumInputPorts=3
      settings: ActiveDisplayString=3  ActiveDisplayYMinimum=-277.52426971765277  ActiveDisplayYMaximum=517.46942172127433  YLabel=Current Phase C
  I_D : Scope  NumInputPorts=2
      settings: ActiveDisplayYMinimum=-1  ActiveDisplayYMaximum=1  YLabel=ID Reference  DataLoggingVariableName=ScopeData4
  I_Q : Scope  NumInputPorts=2
      settings: ActiveDisplayYMinimum=-96.146266364445651  ActiveDisplayYMaximum=95.78745001145893  YLabel=IQ Measured  DataLoggingVariableName=ScopeData3
  Mux : Mux  Inputs=2
  Mux1 : Mux  Inputs=2
  Mux2 : Mux  Inputs=2
  Speed_Torque : Scope  NumInputPorts=3
      settings: ActiveDisplayString=3  ActiveDisplayYMinimum=-31.249999999999638  ActiveDisplayYMaximum=281.24999999999682  YLabel=Torque (Nm)
  Switch : Scope  NumInputPorts=3
      settings: ActiveDisplayString=3  ActiveDisplayYMinimum=-0.12499999999999997  ActiveDisplayYMaximum=1.125  YLabel=Switch C  DataLoggingVariableName=ScopeData2
  wires:
  [speed_ref] -> Speed_Torque/1  "Speed_Reference"
  [Speed_orginal] -> Speed_Torque/2  "Speed_Measured"
  Mux2/1 -> Switch/3  "Switch C"
  [S_CL] -> Mux2/2  "S_CL"
  [S_BH] -> Mux1/1  "S_BH"
  [S_BL] -> Mux1/2  "S_BL"
  Mux/1 -> Switch/1  "Switch A"
  [S_AL] -> Mux/2  "S_AL"
  Mux1/1 -> Switch/2  "Switch B"
  [S_CH] -> Mux2/1  "S_CH"
  [S_AH] -> Mux/1  "S_AH"
  [Torque_measured] -> Speed_Torque/3  "Torque_Measured"
  [Ib_meas] -> Current_ABC/2  "I_B_Measured"
  [Ia_meas] -> Current_ABC/1  "I_A_Measured"
  [Ic_meas] -> Current_ABC/3  "I_C_Measured"
  [id_ref] -> I_D/1  "I_d Reference"
  [id_meas] -> I_D/2  "I_d Measured"
  [iq_ref] -> I_Q/1  "I_q Reference"
  [iq_meas] -> I_Q/2  "I_q Measured"

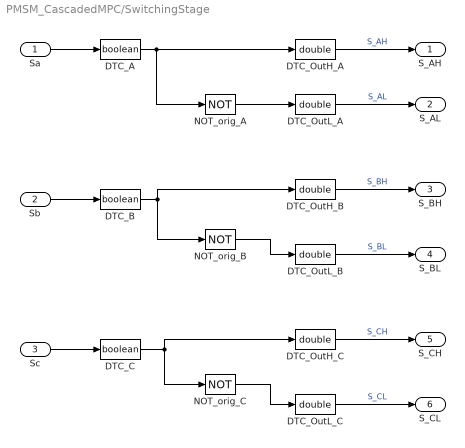
== system PMSM_CascadedMPC/SwitchingStage ==
  Sa : Inport  SampleTime=Ts_sim
  Sb : Inport  Port=2  SampleTime=Ts_sim
  Sc : Inport  Port=3  SampleTime=Ts_sim
  DTC_A : DataTypeConversion  OutDataTypeStr=boolean  SampleTime=Ts_sim  SaturateOnIntegerOverflow=off  RndMeth=Floor
  DTC_B : DataTypeConversion  OutDataTypeStr=boolean  SampleTime=Ts_sim  SaturateOnIntegerOverflow=off  RndMeth=Floor
  DTC_C : DataTypeConversion  OutDataTypeStr=boolean  SampleTime=Ts_sim  SaturateOnIntegerOverflow=off  RndMeth=Floor
  DTC_OutH_A : DataTypeConversion  OutDataTypeStr=double  SampleTime=Ts_sim  SaturateOnIntegerOverflow=off  RndMeth=Floor
  DTC_OutH_B : DataTypeConversion  OutDataTypeStr=double  SampleTime=Ts_sim  SaturateOnIntegerOverflow=off  RndMeth=Floor
  DTC_OutH_C : DataTypeConversion  OutDataTypeStr=double  SampleTime=Ts_sim  SaturateOnIntegerOverflow=off  RndMeth=Floor
  DTC_OutL_A : DataTypeConversion  OutDataTypeStr=double  SampleTime=Ts_sim  SaturateOnIntegerOverflow=off  RndMeth=Floor
  DTC_OutL_B : DataTypeConversion  OutDataTypeStr=double  SampleTime=Ts_sim  SaturateOnIntegerOverflow=off  RndMeth=Floor
  DTC_OutL_C : DataTypeConversion  OutDataTypeStr=double  SampleTime=Ts_sim  SaturateOnIntegerOverflow=off  RndMeth=Floor
  NOT_orig_A : Logic  Operator=NOT  AllPortsSameDT=off  OutDataTypeStr=boolean  SampleTime=Ts_sim
  NOT_orig_B : Logic  Operator=NOT  AllPortsSameDT=off  OutDataTypeStr=boolean  SampleTime=Ts_sim
  NOT_orig_C : Logic  Operator=NOT  AllPortsSameDT=off  OutDataTypeStr=boolean  SampleTime=Ts_sim
  S_AH : Outport  SampleTime=Ts_sim
  S_AL : Outport  Port=2  SampleTime=Ts_sim
  S_BH : Outport  Port=3  SampleTime=Ts_sim
  S_BL : Outport  Port=4  SampleTime=Ts_sim
  S_CH : Outport  Port=5  SampleTime=Ts_sim
  S_CL : Outport  Port=6  SampleTime=Ts_sim
  wires:
  Sa/1 -> DTC_A/1
  DTC_A/1 -> DTC_OutH_A/1, NOT_orig_A/1
  NOT_orig_A/1 -> DTC_OutL_A/1
  DTC_OutH_A/1 -> S_AH/1  "S_AH"
  DTC_OutL_A/1 -> S_AL/1  "S_AL"
  Sb/1 -> DTC_B/1
  DTC_B/1 -> DTC_OutH_B/1, NOT_orig_B/1
  NOT_orig_B/1 -> DTC_OutL_B/1
  DTC_OutH_B/1 -> S_BH/1  "S_BH"
  DTC_OutL_B/1 -> S_BL/1  "S_BL"
  Sc/1 -> DTC_C/1
  DTC_C/1 -> DTC_OutH_C/1, NOT_orig_C/1
  NOT_orig_C/1 -> DTC_OutL_C/1
  DTC_OutH_C/1 -> S_CH/1  "S_CH"
  DTC_OutL_C/1 -> S_CL/1  "S_CL"
